simulink model "Planar_PIDC"  (R2022b)
settings: Solver=VariableStepAuto  StartTime=0.0  StopTime=40  RelTol=1e-3
values from neighbouring files (symbols this model uses):
  I = [1; 1; 1; 0.5; 0.5]*0.2    [RobDyn4link.m]
  l = [1; 1; 1; 1; 2]*0.2    [RobDyn4link.m]
  lc = l./2    [RobDyn4link.m]
  m = [1; 1; 1; 0.3; 0.3]*1    [RobDyn4link.m]
  q0 = [pi/2; -pi/4; -1*pi/6;-pi/12;0;]    [RobDyn4link.m]
  theta_max = [0.915*pi; 0.915*pi; 0.915*pi; 0.915*pi; 0.915*pi;]    [RobDyn4link.m]
  theta_min = [-0.915*pi; -0.915*pi; -0.915*pi; -0.915*pi; -0.915*pi;]    [RobDyn4link.m]
undefined symbols (not defined in the file or in its folder): DiscIntNeverNeededParam
(part 1 of 3)
settings Model: Creator=yu  LastModifiedBy=yu

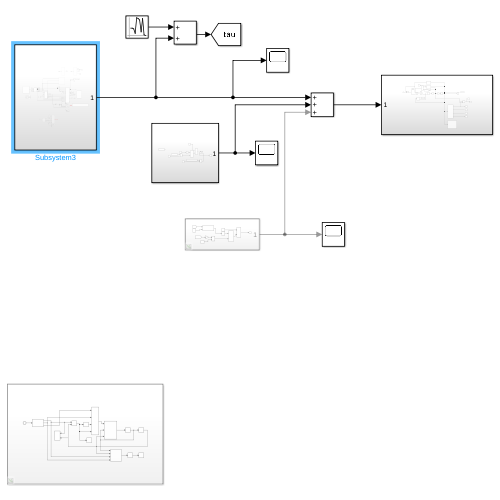
[thumbnail: Simulink's stored preview of the top-level diagram]
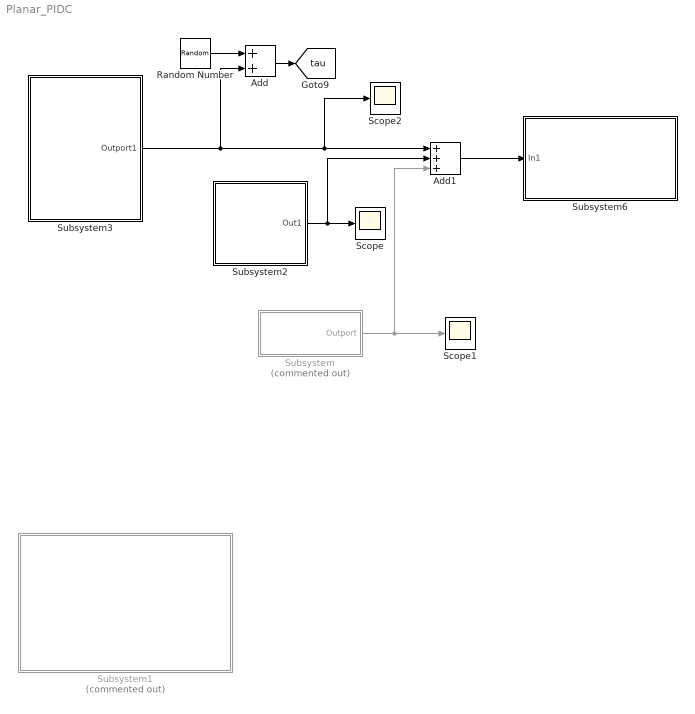
== system Planar_PIDC ==
  Add : Sum
  Add1 : Sum  Inputs=+++
  Random Number : RandomNumber  Variance=0.1
  Scope : Scope
  Scope1 : Scope
  Scope2 : Scope
  Subsystem : Subsystem  Commented=on
  Subsystem1 : Subsystem  Commented=on
  Subsystem2 : Subsystem
  Subsystem3 : Subsystem
  Subsystem6 : Subsystem
  tag scope: tau=global
  wires:
  Add1/1 -> Subsystem6/1(In1)
  Subsystem3/1(Outport1) -> Scope2/1, Add1/1, Add/2
  Subsystem2/1(Out1) -> Scope/1, Add1/2
  Subsystem/1(Outport) -> Scope1/1, Add1/3
  Random Number/1 -> Add/1
  Add/1 -> [tau]

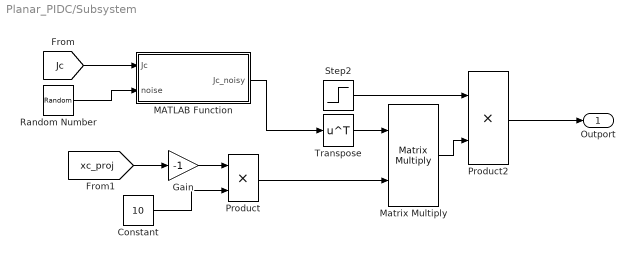
== system Planar_PIDC/Subsystem ==
  Constant : Constant  Value=10
  Gain : Gain  Gain=-1
  MATLAB Function : MATLAB Function  TreatAsAtomicUnit=on
  Matrix Multiply : Product  Multiplication=Matrix(*)
  Product : Product
  Product2 : Product
  Random Number : RandomNumber  SampleTime=0.1
  Step2 : Step  Time=5  After=5  SampleTime=0
  Transpose : Math  Operator=transpose
  Outport : Outport
  wires:
  Step2/1 -> Product2/1
  Matrix Multiply/1 -> Product2/2
  Transpose/1 -> Matrix Multiply/1
  [xc_proj] -> Gain/1
  Product/1 -> Matrix Multiply/2
  Product2/1 -> Outport/1
  [Jc] -> MATLAB Function/1(Jc)
  Constant/1 -> Product/2
  Random Number/1 -> MATLAB Function/2(noise)
  MATLAB Function/1(Jc_noisy) -> Transpose/1
  Gain/1 -> Product/1

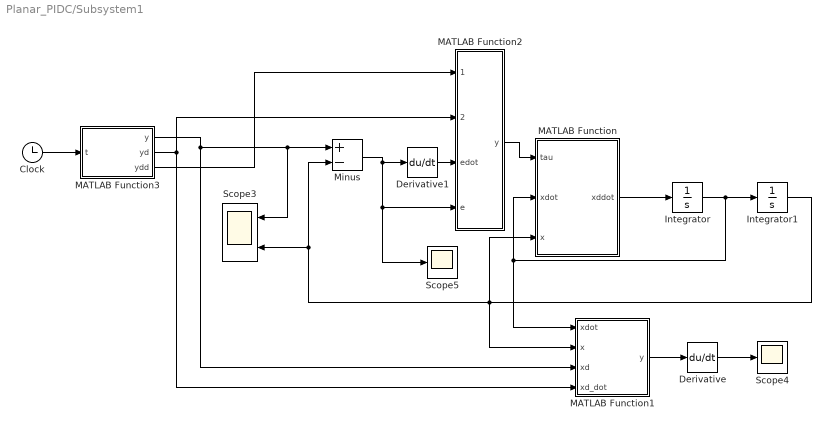
== system Planar_PIDC/Subsystem1 ==
  Clock : Clock
  Derivative : Derivative
  Derivative1 : Derivative
  Integrator : Integrator
  Integrator1 : Integrator
  MATLAB Function : MATLAB Function  TreatAsAtomicUnit=on
  MATLAB Function1 : MATLAB Function  TreatAsAtomicUnit=on
  MATLAB Function2 : MATLAB Function  TreatAsAtomicUnit=on
  MATLAB Function3 : MATLAB Function  TreatAsAtomicUnit=on
  Minus : Sum  Inputs=+-
  Scope3 : Scope  NumInputPorts=2
  Scope4 : Scope
  Scope5 : Scope
  wires:
  Derivative/1 -> Scope4/1
  MATLAB Function3/1(y) -> Scope3/1, Minus/1, MATLAB Function1/3(xd)
  MATLAB Function1/1(y) -> Derivative/1
  MATLAB Function/1(xddot) -> Integrator/1
  Integrator1/1 -> MATLAB Function1/2(x), Minus/2, Scope3/2, MATLAB Function/3(x)
  MATLAB Function2/1(y) -> MATLAB Function/1(tau)
  Clock/1 -> MATLAB Function3/1(t)
  Integrator/1 -> MATLAB Function/2(xdot), MATLAB Function1/1(xdot), Integrator1/1
  Minus/1 -> Scope5/1, MATLAB Function2/4(e), Derivative1/1
  MATLAB Function3/3(ydd) -> MATLAB Function2/1(xd_ddot)
  Derivative1/1 -> MATLAB Function2/3(edot)
  MATLAB Function3/2(yd) -> MATLAB Function2/2(xd_dot), MATLAB Function1/4(xd_dot)

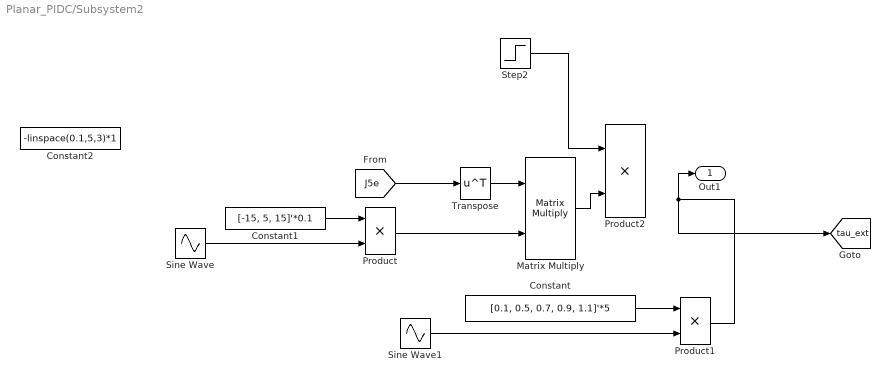
== system Planar_PIDC/Subsystem2 ==
  Constant : Constant  Value=[0.1, 0.5, 0.7, 0.9, 1.1]'*5
  Constant1 : Constant  Value=[-15, 5, 15]'*0.1
  Constant2 : Constant  Value=-linspace(0.1,5,3)*1
  Matrix Multiply : Product  Multiplication=Matrix(*)
  Product : Product
  Product1 : Product
  Product2 : Product
  Sine Wave : Sin  Frequency=0.5  SampleTime=0
  Sine Wave1 : Sin  Frequency=0.5  SampleTime=0
  Step2 : Step  Time=5  After=5  SampleTime=0
  Transpose : Math  Operator=transpose
  Out1 : Outport
  tag scope: tau_ext=global
  wires:
  [J5e] -> Transpose/1
  Transpose/1 -> Matrix Multiply/1
  Product/1 -> Matrix Multiply/2
  Matrix Multiply/1 -> Product2/2
  Product1/1 -> Out1/1, [tau_ext]
  Step2/1 -> Product2/1
  Constant1/1 -> Product/1
  Sine Wave/1 -> Product/2
  Constant/1 -> Product1/1
  Sine Wave1/1 -> Product1/2

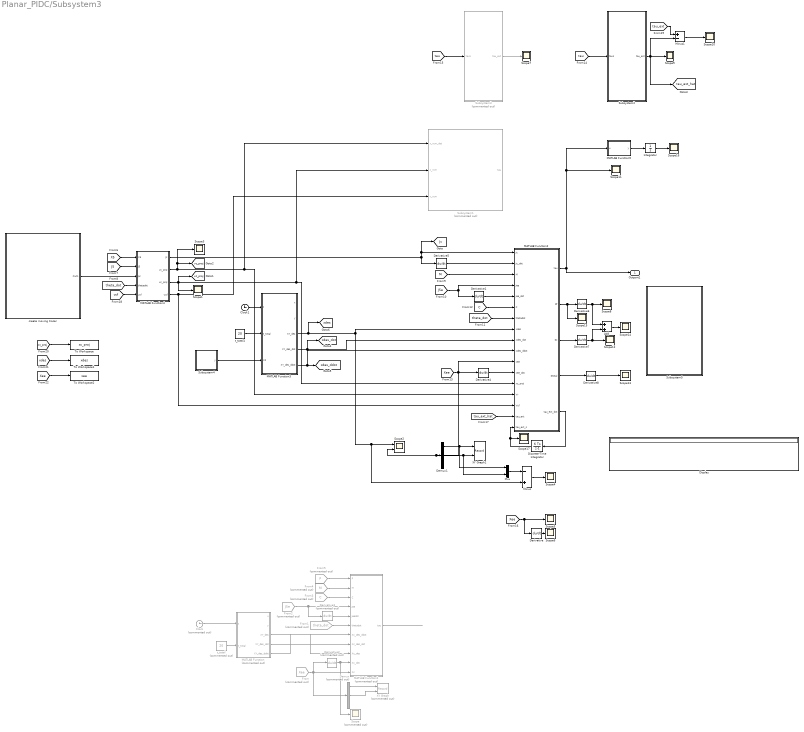
== system Planar_PIDC/Subsystem3 ==
  Add : Sum
  Clock : Clock  Commented=on
  Clock1 : Clock
  Demux : Demux  Commented=on  Outputs=3
  Demux1 : Demux  Outputs=3
  Derivative{,1,4..8} (7 alike) : Derivative
  Derivative2 : Derivative  Commented=on
  Derivative3 : Derivative  Commented=on
  Discrete-Time Integrator : DiscreteIntegrator  SampleTime=1e-3  ICPrevOutput=DiscIntNeverNeededParam  ICPrevScaledInput=DiscIntNeverNeededParam
  Display : Display
  From : From  Commented=on  GotoTag=Xee  TagVisibility=global
  From1 : From  Commented=on  GotoTag=theta_dot  TagVisibility=global
  From2 : From  Commented=on  GotoTag=J5e  TagVisibility=global
  From3 : From  Commented=on  GotoTag=C  TagVisibility=global
  From4 : From  Commented=on  GotoTag=M  TagVisibility=global
  From5 : From  Commented=on  GotoTag=P  TagVisibility=global
  Integrator : Integrator
  MATLAB Function : MATLAB Function  Commented=on  TreatAsAtomicUnit=on
  MATLAB Function1 : MATLAB Function  Commented=on  TreatAsAtomicUnit=on
  MATLAB Function2 : MATLAB Function  TreatAsAtomicUnit=on
  MATLAB Function3 : MATLAB Function  TreatAsAtomicUnit=on
  MATLAB Function4 : MATLAB Function  TreatAsAtomicUnit=on
  MATLAB Function5 : MATLAB Function  TreatAsAtomicUnit=on
  Minus : Sum  Inputs=-+
  Minus1 : Sum  Inputs=+-
  Mux : Mux  Inputs=2
  Scope : Scope  Commented=on
  Scope{1,3..17} (16 alike) : Scope
  Scope2 : Scope  NumInputPorts=2
  Subsystem1 : Subsystem  Commented=on
  Subsystem2 : Subsystem
  Subsystem3 : Subsystem  Commented=on
  Subsystem4 : Subsystem
  Subsystem5 : Subsystem
  To Workspace : ToWorkspace  VariableName=xc_proj  SaveFormat=Timeseries  SampleTime=-1
  To Workspace1 : ToWorkspace  VariableName=xdes  SaveFormat=Timeseries  SampleTime=-1
  To Workspace2 : ToWorkspace  VariableName=xee  SaveFormat=Timeseries  SampleTime=-1
  XY Graph : Record  Commented=on  FileSettingsInternal="{\"entries\":[{\"content\":{\"excelSettings\":{\"content\":{},\"type\":\"Streamout.ExcelSettings\"}},\"type\":\"Streamout.FileSettingStorage\",\"uuid\":\"\"}],\"packageUris\":[\"http:\\/\\/schema.mathworks.com\\/mf0\\/streamout_blocks\\/R2020a\"],\"version\":\"1.0\"}"  Layout=[1 1]  SignalsInternal="{\"entries\":[{\"content\":{\"signals\":[{\"content\":{\"blockPath\":[],\"channel\":[],\"dimensions\":[1,1],\"domain\":\"\",\"lineColor\":\"#a2142f\",\"plots\":[1],\"port\":1,\"sid\":[],\"signalID\":16,\"signalName\":\"Demux:1\"},\"type\":\"RecordBlkView.Signal\",\"uuid\":\"\"},{\"content\":{\"blockPath\":[],\"channel\":[],\"dimensions\":[1,1],\"domain\":\"\",\"lineColor\":\"#139fff\",\"plots\":[1],\"port\":2,\"sid\":[],\"signalID\":19,\"signalName\":\"Demux:2\"},\"type\":\"RecordBlkView.Signal\",\"uuid\":\"\"}]},\"type\":\"RecordBlkView.InputSignals\",\"uuid\":\"\"}],\"packageUris\":[\"http:\\/\\/schema.mathworks.com\\/mf0\\/streamout_blocks\\/R2020a\"],\"version\":\"1.0\"}"  VisualizationBindings="{\"xyplotplugin\":{\"info\":[{\"series\":[{\"bindingParametersList\":[{\"parameter\":\"X-Axis\",\"signalID\":16,\"signalName\":\"Demux:1\"},{\"parameter\":\"Y-Axis\",\"signalID\":19,\"signalName\":\"Demux:2\"}],\"seriesID\":63717}],\"subplotID\":1}]}}"  CompatibilityTag=XY
  XY Graph1 : Record  FileSettingsInternal="{\"entries\":[{\"content\":{\"excelSettings\":{\"content\":{},\"type\":\"Streamout.ExcelSettings\"}},\"type\":\"Streamout.FileSettingStorage\",\"uuid\":\"\"}],\"packageUris\":[\"http:\\/\\/schema.mathworks.com\\/mf0\\/streamout_blocks\\/R2020a\"],\"version\":\"1.0\"}"  Layout=[1 1]  SignalsInternal="{\"entries\":[{\"content\":{\"signals\":[{\"content\":{\"blockPath\":[],\"channel\":[],\"dimensions\":[1,1],\"domain\":\"\",\"lineColor\":\"#a2142f\",\"plots\":[1],\"port\":1,\"sid\":[\"\"],\"signalID\":6665,\"signalName\":\"Demux1:1\"},\"type\":\"RecordBlkView.Signal\",\"uuid\":\"\"},{\"content\":{\"blockPath\":[],\"channel\":[],\"dimensions\":[1,1],\"domain\":\"\",\"lineColor\":\"#139fff\",\"plots\":[1],\"port\":2,\"sid\":[\"\"],\"signalID\":6669,\"signalName\":\"Demux1:2\"},\"type\":\"RecordBlkView.Signal\",\"uuid\":\"\"}]},\"type\":\"RecordBlkView.InputSignals\",\"uuid\":\"\"}],\"packageUris\":[\"http:\\/\\/schema.mathworks.com\\/mf0\\/streamout_blocks\\/R2020a\"],\"version\":\"1.0\"}"  VisualizationBindings="{\"xyplotplugin\":{\"info\":[{\"series\":[{\"bindingParametersList\":[{\"parameter\":\"X-Axis\",\"signalID\":6665,\"signalName\":\"Demux1:1\"},{\"parameter\":\"Y-Axis\",\"signalID\":6669,\"signalName\":\"Demux1:2\"}],\"seriesID\":65386}],\"subplotID\":1}]}}"  CompatibilityTag=XY
  create moving trocar : Subsystem
  t_total : Constant  Commented=on  Value=20
  t_total1 : Constant  Value=20
  Outport1 : Outport
  tag scope: Jc=global, tau_ext_hat=global, vc_proj=global, xc_proj=global, xdes=global, xdes_ddot=global, xdes_dot=global
  wires:
  Clock/1 -> MATLAB Function/1(t)
  t_total/1 -> MATLAB Function/2(t_total)
  MATLAB Function/5(XY_des_ddot) -> MATLAB Function1/7(Xc_des_ddot)
  From/1 -> Demux/1, Derivative2/1, MATLAB Function1/11(Xc)
  Derivative2/1 -> Scope/1, MATLAB Function1/10(Xc_dot)
  From1/1 -> MATLAB Function1/6(thetadot)
  From2/1 -> Derivative3/1, MATLAB Function1/4(Jee)
  Derivative3/1 -> MATLAB Function1/5(Jeedot)
  From3/1 -> MATLAB Function1/3(C)
  From4/1 -> MATLAB Function1/2(M)
  From5/1 -> MATLAB Function1/1(P)
  MATLAB Function1/1(tau) -> ?
  MATLAB Function/3(XY_des) -> MATLAB Function1/9(Xc_des)
  MATLAB Function/4(XY_des_dot) -> MATLAB Function1/8(Xc_des_dot)
  Demux/1 -> XY Graph/1
  Demux/2 -> XY Graph/2
  [X5] -> MATLAB Function4/1(X5)
  [theta_dot] -> MATLAB Function4/4(thetadot)
  [J5] -> MATLAB Function4/2(J5)
  [M] -> MATLAB Function2/3(M)
  Derivative1/1 -> MATLAB Function2/5(Jee_dot)
  [J5e] -> MATLAB Function2/4(Jee), Derivative1/1
  [theta_dot] -> MATLAB Function2/7(thetadot)
  [C] -> MATLAB Function2/6(C)
  [Xee] -> Derivative4/1, Scope2/2, Demux1/1, MATLAB Function2/11(xee)
  Derivative4/1 -> MATLAB Function2/12(xee_dot)
  Demux1/1 -> Mux/1, XY Graph1/1
  Demux1/2 -> Mux/2, XY Graph1/2
  MATLAB Function4/3(xc_proj) -> MATLAB Function2/13(xc_proj), Subsystem1/2(x_rcm), Scope1/1, [xc_proj]
  MATLAB Function4/2(vc_proj) -> Scope3/1, [vc_proj], MATLAB Function2/14(Vr), Subsystem1/1(x_rcm_dot)
  Mux/1 -> Minus/1
  Minus/1 -> Scope4/1
  [Xee] -> Derivative/1, Scope5/1
  Derivative/1 -> Scope6/1
  [vcf] -> MATLAB Function4/5(vcf)
  create moving trocar/1(Out1) -> MATLAB Function4/3(pc)
  Derivative5/1 -> MATLAB Function2/2(Jc_dot)
  MATLAB Function4/4(Vcf) -> Subsystem1/3(v_rcm), MATLAB Function2/15(Vcf)
  MATLAB Function4/1(Jc) -> [Jc], MATLAB Function2/1(Jc), Derivative5/1
  [tau] -> Subsystem2/1(tau1)
  Subsystem2/1(tau_ext) -> [tau_ext_hat], Scope9/1, Minus1/2
  Subsystem3/1(tau_ext) -> Scope7/1
  [tau] -> Subsystem3/1(tau1)
  MATLAB Function3/3(XY_des) -> Minus/2, Scope2/1, MATLAB Function2/8(xdes), [xdes]
  MATLAB Function3/4(XY_des_dot) -> MATLAB Function2/9(xdes_dot), [xdes_dot]
  MATLAB Function3/5(XY_des_ddot) -> MATLAB Function2/10(xdes_ddot), [xdes_ddot]
  [tau_ext_hat] -> MATLAB Function2/16(tau_ext)
  [tau_ext] -> Minus1/1
  Minus1/1 -> Scope10/1
  Clock1/1 -> MATLAB Function3/1(t)
  t_total1/1 -> MATLAB Function3/2(t_total)
  Subsystem4/1(y) -> MATLAB Function3/3(X0)
  MATLAB Function2/2(Sf) -> Scope15/1, Derivative6/1
  MATLAB Function2/3(Sc) -> Derivative7/1
  Derivative6/1 -> Add/1, Scope8/1
  Derivative7/1 -> Add/2, Scope12/1
  MATLAB Function2/4(Stotal) -> Derivative8/1
  Derivative8/1 -> Scope13/1
  Add/1 -> Scope14/1
  MATLAB Function2/1(tau) -> Outport1/1, Scope11/1, MATLAB Function5/1(u)
  MATLAB Function5/1(y) -> Integrator/1
  Integrator/1 -> Scope16/1
  [xc_proj] -> To Workspace/1
  [xdes] -> To Workspace1/1
  [Xee] -> To Workspace2/1
  Discrete-Time Integrator/1 -> Scope17/1, MATLAB Function2/17(tau_ext_s)
  MATLAB Function2/5(tau_ext_dot) -> Discrete-Time Integrator/1

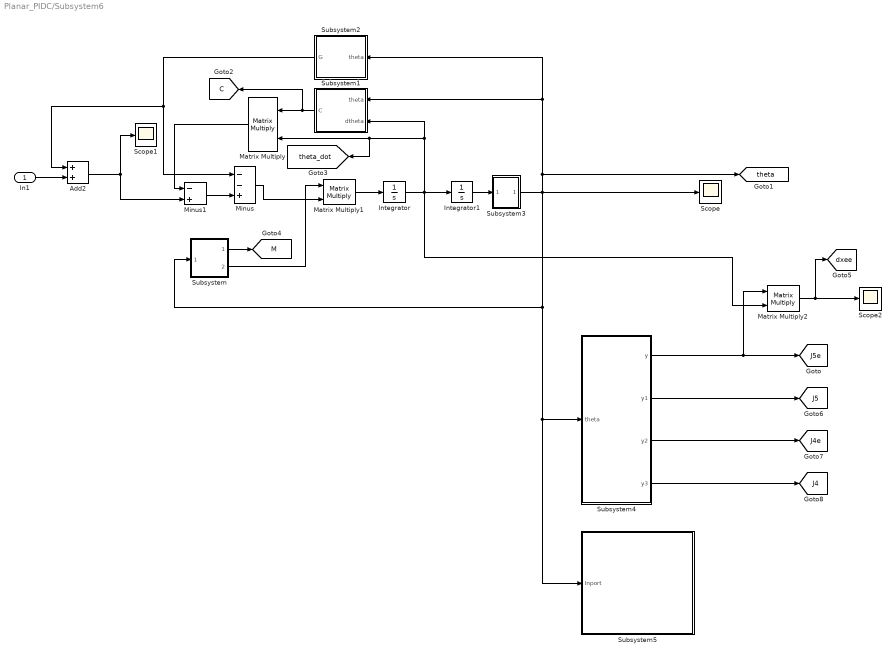
== system Planar_PIDC/Subsystem6 ==
  In1 : Inport
  Add2 : Sum
  Integrator : Integrator
  Integrator1 : Integrator  InitialCondition=q0
  Matrix Multiply : Product  Multiplication=Matrix(*)
  Matrix Multiply1 : Product  Multiplication=Matrix(*)
  Matrix Multiply2 : Product  Multiplication=Matrix(*)
  Minus : Sum  Inputs=--+
  Minus1 : Sum  Inputs=-+
  Scope : Scope
  Scope1 : Scope
  Scope2 : Scope
  Subsystem : Subsystem
  Subsystem1 : Subsystem
  Subsystem2 : Subsystem
  Subsystem3 : Subsystem
  Subsystem4 : Subsystem
  Subsystem5 : Subsystem
  tag scope: C=global, J4=global, J4e=global, J5=global, J5e=global, M=global, dxee=global, theta=global, theta_dot=global
  wires:
  Subsystem2/1(G) -> Minus/1, Add2/1
  Subsystem/2(Outport1) -> Matrix Multiply1/1
  Subsystem/1(Outport) -> [M]
  In1/1 -> Add2/2
  Integrator1/1 -> Subsystem3/1(In1)
  Integrator/1 -> Matrix Multiply2/2, Integrator1/1, Subsystem1/2(dtheta), Matrix Multiply/2, [theta_dot]
  Subsystem4/2(y1) -> [J5]
  Subsystem4/4(y3) -> [J4]
  Matrix Multiply/1 -> Minus1/1
  Add2/1 -> Minus1/2, Scope1/1
  Subsystem4/3(y2) -> [J4e]
  Subsystem3/1(theta) -> Subsystem4/1(theta), Subsystem5/1(Inport), Subsystem/1(Inport), Subsystem1/1(theta), Subsystem2/1(theta), [theta], Scope/1
  Matrix Multiply1/1 -> Integrator/1
  Subsystem4/1(y) -> [J5e], Matrix Multiply2/1
  Subsystem1/1(C) -> [C], Matrix Multiply/1
  Minus/1 -> Matrix Multiply1/2
  Matrix Multiply2/1 -> Scope2/1, [dxee]
  Minus1/1 -> Minus/3

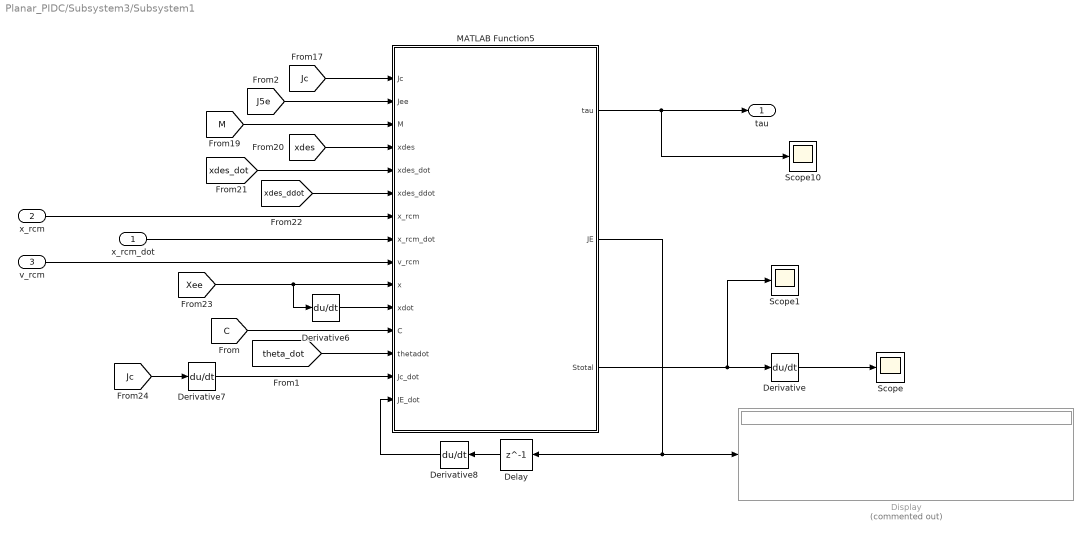
== system Planar_PIDC/Subsystem3/Subsystem1 ==
  x_rcm_dot : Inport
  x_rcm : Inport  Port=2
  v_rcm : Inport  Port=3
  Delay : Delay  DelayLength=1
  Derivative{,6..8} (4 alike) : Derivative
  Display : Display  Commented=on
  MATLAB Function5 : MATLAB Function  TreatAsAtomicUnit=on
  Scope : Scope
  Scope1 : Scope
  Scope10 : Scope
  tau : Outport
  wires:
  [xdes_dot] -> MATLAB Function5/5(xdes_dot)
  [Jc] -> MATLAB Function5/1(Jc)
  [xdes_ddot] -> MATLAB Function5/6(xdes_ddot)
  Derivative6/1 -> MATLAB Function5/11(xdot)
  v_rcm/1 -> MATLAB Function5/9(v_rcm)
  x_rcm/1 -> MATLAB Function5/7(x_rcm)
  [theta_dot] -> MATLAB Function5/13(thetadot)
  x_rcm_dot/1 -> MATLAB Function5/8(x_rcm_dot)
  Derivative7/1 -> MATLAB Function5/14(Jc_dot)
  Derivative8/1 -> MATLAB Function5/15(JE_dot)
  [C] -> MATLAB Function5/12(C)
  [Xee] -> Derivative6/1, MATLAB Function5/10(x)
  [xdes] -> MATLAB Function5/4(xdes)
  [Jc] -> Derivative7/1
  [M] -> MATLAB Function5/3(M)
  MATLAB Function5/2(JE) -> Delay/1, Display/1
  Delay/1 -> Derivative8/1
  MATLAB Function5/1(tau) -> Scope10/1, tau/1
  [J5e] -> MATLAB Function5/2(Jee)
  Derivative/1 -> Scope/1
  MATLAB Function5/3(Stotal) -> Scope1/1, Derivative/1

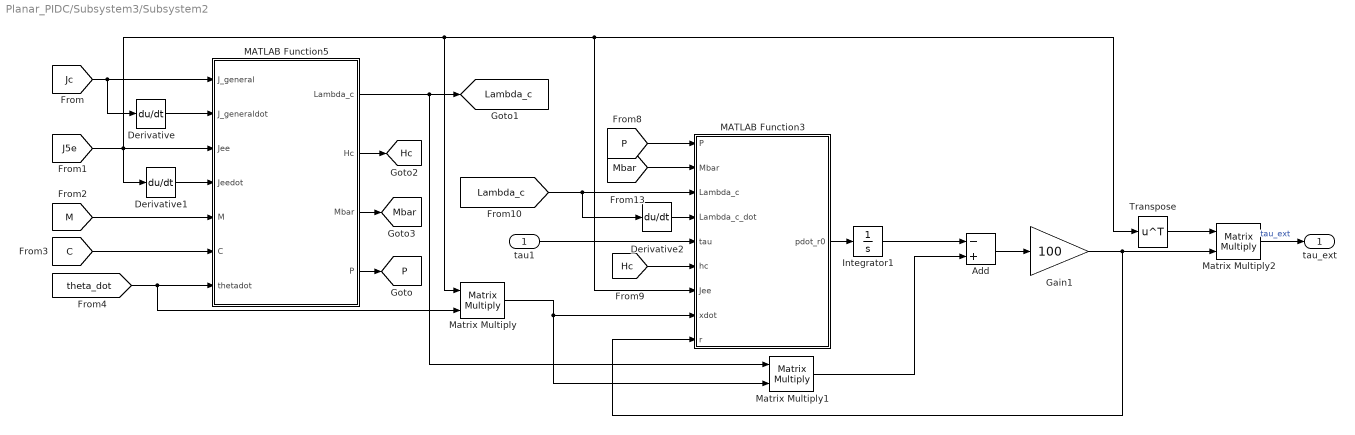
== system Planar_PIDC/Subsystem3/Subsystem2 ==
  tau1 : Inport
  Add : Sum  Inputs=-+
  Derivative : Derivative
  Derivative1 : Derivative
  Derivative2 : Derivative
  Gain1 : Gain  Gain=100
  Integrator1 : Integrator
  MATLAB Function3 : MATLAB Function  TreatAsAtomicUnit=on
  MATLAB Function5 : MATLAB Function  TreatAsAtomicUnit=on
  Matrix Multiply : Product  Multiplication=Matrix(*)
  Matrix Multiply1 : Product  Multiplication=Matrix(*)
  Matrix Multiply2 : Product  Multiplication=Matrix(*)
  Transpose : Math  Operator=transpose
  tau_ext : Outport
  tag scope: Hc=global, Lambda_c=global, Mbar=global, P=global
  wires:
  Matrix Multiply1/1 -> Add/2
  Derivative1/1 -> MATLAB Function5/4(Jeedot)
  MATLAB Function5/1(Lambda_c) -> [Lambda_c], Matrix Multiply1/1
  Gain1/1 -> Matrix Multiply2/2, MATLAB Function3/9(r)
  [J5e] -> MATLAB Function3/7(Jee), Transpose/1, Matrix Multiply/1, MATLAB Function5/3(Jee), Derivative1/1
  tau1/1 -> MATLAB Function3/5(tau)
  MATLAB Function5/2(Hc) -> [Hc]
  Matrix Multiply2/1 -> tau_ext/1  "tau_ext"
  [Lambda_c] -> Derivative2/1, MATLAB Function3/3(Lambda_c)
  Derivative/1 -> MATLAB Function5/2(J_generaldot)
  Integrator1/1 -> Add/1
  MATLAB Function3/1(pdot_r0) -> Integrator1/1
  [C] -> MATLAB Function5/6(C)
  [Hc] -> MATLAB Function3/6(hc)
  MATLAB Function5/3(Mbar) -> [Mbar]
  Matrix Multiply/1 -> MATLAB Function3/8(xdot), Matrix Multiply1/2
  Derivative2/1 -> MATLAB Function3/4(Lambda_c_dot)
  MATLAB Function5/4(P) -> [P]
  [Mbar] -> MATLAB Function3/2(Mbar)
  [P] -> MATLAB Function3/1(P)
  Transpose/1 -> Matrix Multiply2/1
  [theta_dot] -> Matrix Multiply/2, MATLAB Function5/7(thetadot)
  [Jc] -> Derivative/1, MATLAB Function5/1(J_general)
  [M] -> MATLAB Function5/5(M)
  Add/1 -> Gain1/1

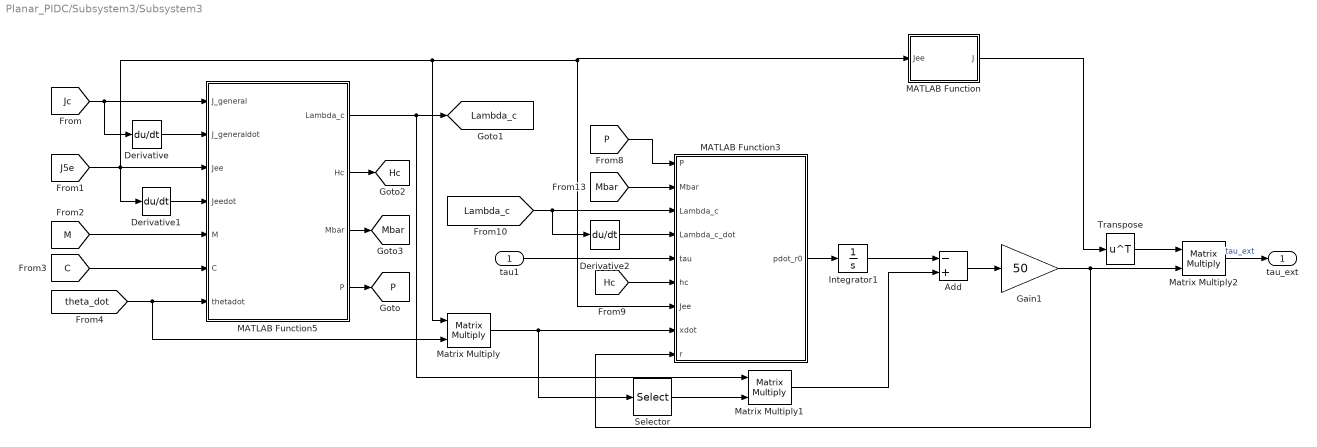
== system Planar_PIDC/Subsystem3/Subsystem3 ==
  tau1 : Inport
  Add : Sum  Inputs=-+
  Derivative : Derivative
  Derivative1 : Derivative
  Derivative2 : Derivative
  Gain1 : Gain  Gain=50
  Integrator1 : Integrator
  MATLAB Function : MATLAB Function  TreatAsAtomicUnit=on
  MATLAB Function3 : MATLAB Function  TreatAsAtomicUnit=on
  MATLAB Function5 : MATLAB Function  TreatAsAtomicUnit=on
  Matrix Multiply : Product  Multiplication=Matrix(*)
  Matrix Multiply1 : Product  Multiplication=Matrix(*)
  Matrix Multiply2 : Product  Multiplication=Matrix(*)
  Selector : Selector  InputPortWidth=3  IndexOptions=Index vector (dialog)  Indices=[1 2]  OutputSizes=1
  Transpose : Math  Operator=transpose
  tau_ext : Outport
  tag scope: Hc=global, Lambda_c=global, Mbar=global, P=global
  wires:
  Add/1 -> Gain1/1
  [M] -> MATLAB Function5/5(M)
  [Jc] -> MATLAB Function5/1(J_general), Derivative/1
  [theta_dot] -> MATLAB Function5/7(thetadot), Matrix Multiply/2
  Transpose/1 -> Matrix Multiply2/1
  [P] -> MATLAB Function3/1(P)
  [Mbar] -> MATLAB Function3/2(Mbar)
  MATLAB Function5/4(P) -> [P]
  Derivative2/1 -> MATLAB Function3/4(Lambda_c_dot)
  Matrix Multiply/1 -> Selector/1, MATLAB Function3/8(xdot)
  MATLAB Function5/3(Mbar) -> [Mbar]
  [Hc] -> MATLAB Function3/6(hc)
  [C] -> MATLAB Function5/6(C)
  MATLAB Function3/1(pdot_r0) -> Integrator1/1
  Integrator1/1 -> Add/1
  Derivative/1 -> MATLAB Function5/2(J_generaldot)
  [Lambda_c] -> MATLAB Function3/3(Lambda_c), Derivative2/1
  Matrix Multiply2/1 -> tau_ext/1  "tau_ext"
  MATLAB Function5/2(Hc) -> [Hc]
  tau1/1 -> MATLAB Function3/5(tau)
  [J5e] -> Derivative1/1, MATLAB Function5/3(Jee), Matrix Multiply/1, MATLAB Function3/7(Jee), MATLAB Function/1(Jee)
  Gain1/1 -> MATLAB Function3/9(r), Matrix Multiply2/2
  MATLAB Function5/1(Lambda_c) -> Matrix Multiply1/1, [Lambda_c]
  Derivative1/1 -> MATLAB Function5/4(Jeedot)
  Matrix Multiply1/1 -> Add/2
  MATLAB Function/1(J) -> Transpose/1
  Selector/1 -> Matrix Multiply1/2

== system Planar_PIDC/Subsystem3/Subsystem4 ==
  Clock2 : Clock
  Constant : Constant  Value=[4.673;1.966]
  Constant1 : Constant  Value=[0.9346,0.3932]
  Display : Display
  MATLAB Function5 : MATLAB Function  TreatAsAtomicUnit=on
  Memory : Memory
  y : Outport
  wires:
  Clock2/1 -> MATLAB Function5/2(t)
  [Xee] -> MATLAB Function5/1(Xee)
  Memory/1 -> MATLAB Function5/3(y_prev)
  Constant1/1 -> Memory/1, Display/1, y/1

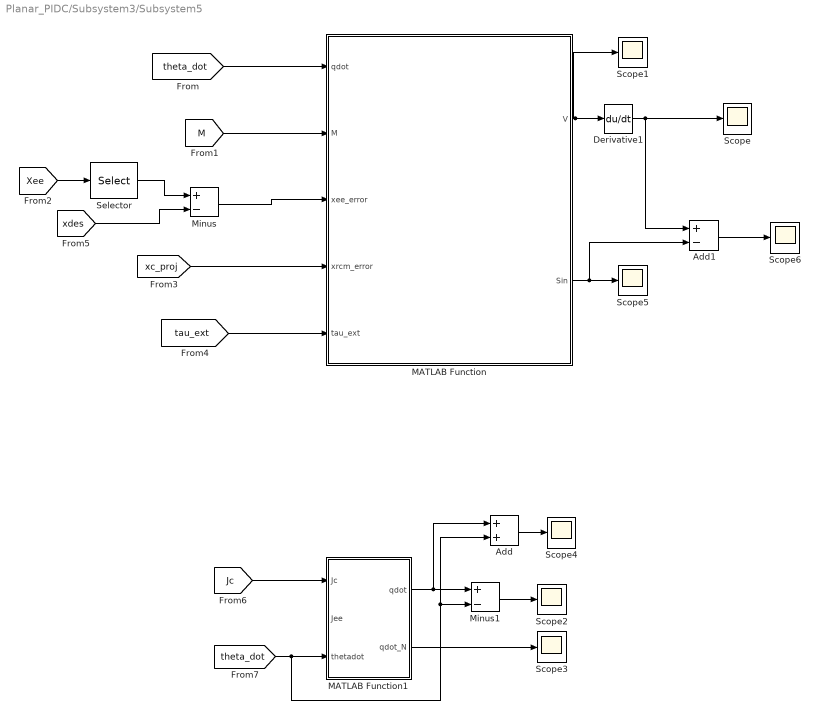
== system Planar_PIDC/Subsystem3/Subsystem5 ==
  Add : Sum
  Add1 : Sum  Inputs=+-
  Derivative1 : Derivative
  MATLAB Function : MATLAB Function  TreatAsAtomicUnit=on
  MATLAB Function1 : MATLAB Function  TreatAsAtomicUnit=on
  Minus : Sum  Inputs=+-
  Minus1 : Sum  Inputs=+-
  Scope{,1..6} (7 alike) : Scope
  Selector : Selector  InputPortWidth=3  IndexOptions=Index vector (dialog)  Indices=[1 2]  OutputSizes=1
  wires:
  [theta_dot] -> MATLAB Function/1(qdot)
  [M] -> MATLAB Function/2(M)
  [xc_proj] -> MATLAB Function/4(xrcm_error)
  [tau_ext] -> MATLAB Function/5(tau_ext)
  Minus/1 -> MATLAB Function/3(xee_error)
  MATLAB Function/1(V) -> Scope1/1, Derivative1/1
  Derivative1/1 -> Add1/1, Scope/1
  Selector/1 -> Minus/1
  [xdes] -> Minus/2
  [Xee] -> Selector/1
  [theta_dot] -> Add/2, Minus1/2, MATLAB Function1/3(thetadot)
  [Jc] -> MATLAB Function1/1(Jc)
  MATLAB Function1/1(qdot) -> Add/1, Minus1/1
  Minus1/1 -> Scope2/1
  MATLAB Function1/2(qdot_N) -> Scope3/1
  Add/1 -> Scope4/1
  MATLAB Function/2(Sin) -> Add1/2, Scope5/1
  Add1/1 -> Scope6/1

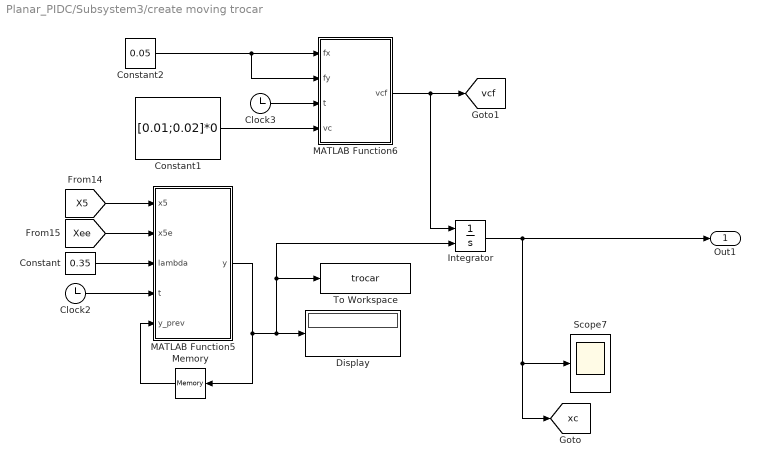
== system Planar_PIDC/Subsystem3/create moving trocar ==
  Clock2 : Clock
  Clock3 : Clock
  Constant : Constant  Value=0.35
  Constant1 : Constant  Value=[0.01;0.02]*0
  Constant2 : Constant  Value=0.05
  Display : Display
  Integrator : Integrator  InitialConditionSource=external
  MATLAB Function5 : MATLAB Function  TreatAsAtomicUnit=on
  MATLAB Function6 : MATLAB Function  TreatAsAtomicUnit=on
  Memory : Memory
  Scope7 : Scope
  To Workspace : ToWorkspace  VariableName=trocar  SaveFormat=Timeseries  SampleTime=-1
  Out1 : Outport
  tag scope: vcf=global, xc=global
  wires:
  Clock3/1 -> MATLAB Function6/3(t)
  [Xee] -> MATLAB Function5/2(x5e)
  Constant2/1 -> MATLAB Function6/2(fy), MATLAB Function6/1(fx)
  Clock2/1 -> MATLAB Function5/4(t)
  [X5] -> MATLAB Function5/1(x5)
  Constant1/1 -> MATLAB Function6/4(vc)
  MATLAB Function6/1(vcf) -> [vcf], Integrator/1
  Constant/1 -> MATLAB Function5/3(lambda)
  Integrator/1 -> Out1/1, [xc], Scope7/1
  Memory/1 -> MATLAB Function5/5(y_prev)
  MATLAB Function5/1(y) -> Memory/1, To Workspace/1, Integrator/2, Display/1

== system Planar_PIDC/Subsystem6/Subsystem ==
  Inport : Inport  PortDimensions=[5,1]
  Constant : Constant  Value=l
  Constant1 : Constant  Value=lc
  Constant2 : Constant  Value=I
  Constant3 : Constant  Value=m
  MATLAB Function : MATLAB Function  TreatAsAtomicUnit=on
  Outport : Outport  PortDimensions=[5,5]
  Outport1 : Outport  Port=2  PortDimensions=[5,5]
  wires:
  Constant3/1 -> MATLAB Function/5(m)
  MATLAB Function/1(M) -> Outport/1  "M"
  Inport/1 -> MATLAB Function/1(theta)  "theta"
  Constant2/1 -> MATLAB Function/4(I)
  Constant/1 -> MATLAB Function/2(l)
  Constant1/1 -> MATLAB Function/3(lc)
  MATLAB Function/2(Minv) -> Outport1/1  "Minv"

== system Planar_PIDC/Subsystem6/Subsystem1 ==
  theta : Inport  PortDimensions=[5,1]
  dtheta : Inport  Port=2  PortDimensions=[5,1]
  Constant : Constant  Value=m
  Constant1 : Constant  Value=l
  Constant2 : Constant  Value=lc
  MATLAB Function : MATLAB Function  TreatAsAtomicUnit=on
  C : Outport  PortDimensions=[5,5]
  wires:
  theta/1 -> MATLAB Function/1(theta)
  MATLAB Function/1(C) -> C/1
  dtheta/1 -> MATLAB Function/2(dtheta)
  Constant/1 -> MATLAB Function/3(m)
  Constant2/1 -> MATLAB Function/5(lc)
  Constant1/1 -> MATLAB Function/4(l)

== system Planar_PIDC/Subsystem6/Subsystem2 ==
  theta : Inport  PortDimensions=[5,1]
  Constant : Constant  Value=m
  Constant1 : Constant  Value=l
  Constant2 : Constant  Value=lc
  MATLAB Function : MATLAB Function  TreatAsAtomicUnit=on
  G : Outport  PortDimensions=[5,1]
  wires:
  Constant1/1 -> MATLAB Function/3(l)
  Constant2/1 -> MATLAB Function/4(lc)
  Constant/1 -> MATLAB Function/2(m)
  MATLAB Function/1(G) -> G/1
  theta/1 -> MATLAB Function/1(theta)

== system Planar_PIDC/Subsystem6/Subsystem3 ==
  In1 : Inport
  Atan2 : Trigonometry  Operator=atan2
  Constant : Constant  Value=theta_max
  Constant1 : Constant  Value=theta_min
  MATLAB Function : MATLAB Function  TreatAsAtomicUnit=on
  Sin : Trigonometry
  Sin1 : Trigonometry  Operator=cos
  theta : Outport  PortDimensions=[5,1]
  wires:
  Atan2/1 -> MATLAB Function/1(theta)
  In1/1 -> Sin1/1, Sin/1
  Sin/1 -> Atan2/1
  Sin1/1 -> Atan2/2
  MATLAB Function/1(y) -> theta/1
  Constant/1 -> MATLAB Function/2(theta_max)
  Constant1/1 -> MATLAB Function/3(theta_min)

== system Planar_PIDC/Subsystem6/Subsystem4 ==
  theta : Inport
  Constant : Constant  Value=l
  MATLAB Function : MATLAB Function  TreatAsAtomicUnit=on
  y : Outport
  y1 : Outport  Port=2
  y2 : Outport  Port=3
  y3 : Outport  Port=4
  wires:
  theta/1 -> MATLAB Function/1(theta)  "theta"
  MATLAB Function/1(J5e) -> y/1  "J5e"
  Constant/1 -> MATLAB Function/2(l)
  MATLAB Function/2(J5) -> y1/1  "J5"
  MATLAB Function/3(J4e) -> y2/1  "J4e"
  MATLAB Function/4(J4) -> y3/1  "J4"

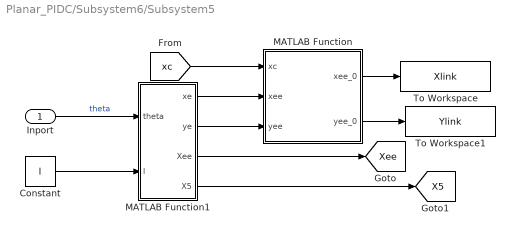
== system Planar_PIDC/Subsystem6/Subsystem5 ==
  Inport : Inport
  Constant : Constant  Value=l
  MATLAB Function : MATLAB Function  TreatAsAtomicUnit=on
  MATLAB Function1 : MATLAB Function  TreatAsAtomicUnit=on
  To Workspace : ToWorkspace  VariableName=Xlink  SaveFormat=Timeseries  SampleTime=-1
  To Workspace1 : ToWorkspace  VariableName=Ylink  SaveFormat=Timeseries  SampleTime=-1
  tag scope: X5=global, Xee=global
  wires:
  MATLAB Function1/1(xe) -> MATLAB Function/2(xee)
  MATLAB Function1/2(ye) -> MATLAB Function/3(yee)
  Inport/1 -> MATLAB Function1/1(theta)  "theta"
  Constant/1 -> MATLAB Function1/2(l)
  MATLAB Function1/3(Xee) -> [Xee]
  MATLAB Function/1(xee_0) -> To Workspace/1
  MATLAB Function/2(yee_0) -> To Workspace1/1
  MATLAB Function1/4(X5) -> [X5]
  [xc] -> MATLAB Function/1(xc)

== matlab function Planar_PIDC/Subsystem6/Subsystem3/MATLAB Function ==
  data: theta input; y output; theta_max input; theta_min input
function y = fcn(theta, theta_max, theta_min)
y= max(theta_min,min(theta, theta_max));

== matlab function Planar_PIDC/Subsystem3/MATLAB Function3 ==
  data: x output; t input; y output; t_total input; XY_des output; XY_des_dot output; XY_des_ddot output; X0 input
function [x,y,XY_des,XY_des_dot,XY_des_ddot]= fcn(t, t_total, X0)
% x0 = 0.934607;
% y0 = 0.393185;

x0 = X0(1);
y0 = X0(2);



radius = 0.05;     % Total duration to complete the circle (seconds)
% dt = 0.01;        % Time step for simulation

% Calculate center of the circle
xc = x0 - radius;
yc = y0;

omega = 2 * pi / t_total;

% Circle trajectory
x = xc + radius * cos(omega * t);
y = yc + radius * sin(omega * t);

% Velocity
xdot = -radius * omega * sin(omega * t);
ydot = radius * omega * cos(omega * t);

% Acceleration
xddot = -radius * omega^2 * cos(omega * t);
yddot = -radius * omega^2 * sin(omega * t);

XY_des = [x;y];
XY_des_dot = [xdot;ydot];
XY_des_ddot = [xddot;yddot];

== matlab function Planar_PIDC/Subsystem3/create moving trocar/MATLAB Function5 ==
  data: x5 input; y output; x5e input; lambda input; t input; y_prev input
function y = fcn(x5,x5e,lambda,t,y_prev)
if t == 0
    xc = lambda*(x5e - x5) + x5;
    y = xc(1:2);
else 
    y = y_prev;
end

== matlab function Planar_PIDC/Subsystem3/create moving trocar/MATLAB Function6 ==
  data: fx input; vcf output; fy input; t input; vc input
function vcf = fcn(fx,fy,t,vc)

vcf = [vc(1)*sin(2*pi*fx*t);
    vc(2)*cos(2*pi*fy*t)];

== matlab function Planar_PIDC/Subsystem3/Subsystem5/MATLAB Function1 ==
  data: Jc input; qdot output; Jee input; thetadot input; qdot_N output
function [qdot,qdot_N]= fcn(Jc,Jee,thetadot)
Jc_pinv = Jc'/(Jc*Jc');
P = eye(5) - Jc_pinv*Jc;
qdot = P*thetadot;
qdot_N = (eye(5) - P)*thetadot;

== matlab function Planar_PIDC/Subsystem3/Subsystem1/MATLAB Function5 ==
  data: Jc input; Jee input; tau output; M input; xdes input; xdes_dot input; xdes_ddot input; x_rcm input; x_rcm_dot input; v_rcm input; x input; xdot input; C input; thetadot input; Jc_dot input; JE_dot input; JE output; Stotal output
function [tau,JE,Stotal]= fcn(Jc,Jee,M,xdes,xdes_dot,xdes_ddot,x_rcm,x_rcm_dot, v_rcm,x,xdot,C,thetadot,Jc_dot,JE_dot)
Jm = Jc(:,1:1);
Jr = Jc(:,2:5);
Z = [-Jr'*inv(Jm)', eye(4)]';
% Z = Z;
Z_sharp = inv(Z'*M*Z)*Z'*M;

Lambda_rcm = inv(Jc/M*Jc');
Lambda_f = Z'*M*Z;
Lambda_E = zeros(5,5);
Lambda_E(1,1) = Lambda_rcm;
Lambda_E(2:5,2:5) = Lambda_f;

JE = [Jc;Z_sharp];

H_E = Lambda_E*(JE/M*C*thetadot - JE_dot*thetadot);

Kp_rcm = 100;
Kd_rcm = sqrt(2)*Kp_rcm;
Frcm = Lambda_rcm * 0 - Kd_rcm*x_rcm_dot - Kp_rcm*x_rcm - v_rcm;

xdes_aug = [xdes];
xdes_dot_aug = [xdes_dot];
xdes_ddot_aug = [xdes_ddot];

Kp = 100;
Kd = sqrt(2)*Kp;
% Kp_matrix = zeros(4,4);
% Kp_matrix(1:2,1:2) = eye(2)*Kp;
Kp_matrix = eye(2)*Kp;
% Kd_matrix = zeros(4,4);
% Kd_matrix(1:2,1:2) = eye(2)*Kd;
Kd_matrix = eye(2)*Kd;

x_aug = [x(1:2)];
xdot_aug = [xdot(1:2)];

Jee = Jee(1:2,:);
Ff =  Lambda_f(1:2,1:2)*xdes_ddot_aug +  Kd_matrix*(xdes_dot_aug - xdot_aug) + Kp_matrix*(xdes_aug - x_aug);
Ff = Z'*Jee'*Ff;

% JE = [Jc; Z_sharp];
tau = JE'*([Frcm;Ff] + H_E);

S = 0.5*((xdes_dot_aug - xdot_aug)'*Lambda_f(1:2,1:2)*(xdes_dot_aug - xdot_aug) + x_rcm_dot'*Lambda_rcm*x_rcm_dot);
V = 0.5*((xdes_aug - x_aug)'*Kp_matrix*(xdes_aug - x_aug) + x_rcm'*Kp_rcm*x_rcm);
Stotal = S + V;

== matlab function Planar_PIDC/Subsystem3/Subsystem4/MATLAB Function5 ==
  data: Xee input; y output; t input; y_prev input
function y = fcn(Xee,t,y_prev)
x0 = zeros(2,1);
if t == 0
    x0 = Xee(1:2);
    y = x0(1:2);
else 
    y = y_prev;
end

== matlab function Planar_PIDC/Subsystem3/MATLAB Function4 ==
  data: X5 input; J5 input; Jc output; vc_proj output; pc input; xc_proj output; thetadot input; vcf input; Vcf output
function [Jc,vc_proj,xc_proj,Vcf] = fcn(X5, J5, pc,thetadot,vcf)
pr = X5(1:2);
theta5 = X5(3);

R = [cos(theta5), -sin(theta5); sin(theta5), cos(theta5)];
y = R(:,2);
dir = pr - pc;
% A = [-y(1), y(2), dir(2)*y(2) - dir(1)*y(1)];
A = [-sin(theta5),cos(theta5),-cos(theta5)*dir(1) - sin(theta5)*dir(2)];
Jc = A*J5;

vc_proj = Jc*thetadot;
xc_proj = R(:,2)'*dir;

Vcf = A(:,1:2)*vcf;

== matlab function Planar_PIDC/Subsystem3/MATLAB Function ==
  data: x output; t input; y output; t_total input; XY_des output; XY_des_dot output; XY_des_ddot output
function [x,y,XY_des,XY_des_dot,XY_des_ddot]= fcn(t, t_total)
x0 = 0.934607;
y0 = 0.393185;

radius = 0.05;     % Total duration to complete the circle (seconds)
% dt = 0.01;        % Time step for simulation

% Calculate center of the circle
xc = x0 - radius;
yc = y0;

omega = 2 * pi / t_total;

% Circle trajectory
x = xc + radius * cos(omega * t);
y = yc + radius * sin(omega * t);

% Velocity
xdot = -radius * omega * sin(omega * t);
ydot = radius * omega * cos(omega * t);

% Acceleration
xddot = -radius * omega^2 * cos(omega * t);
yddot = -radius * omega^2 * sin(omega * t);

XY_des = [x;y];
XY_des_dot = [xdot;ydot];
XY_des_ddot = [xddot;yddot];

== matlab function Planar_PIDC/Subsystem3/MATLAB Function1 ==
  data: P input; tau output; M input; C input; Jee input; Jeedot input; thetadot input; Xc_des_ddot input; Xc_des_dot input; Xc_des input; Xc_dot input; Xc input
function tau = fcn(P, M, C, Jee, Jeedot, thetadot, Xc_des_ddot, Xc_des_dot, Xc_des, Xc_dot, Xc)

% Compute pseudo-inverse of Jee
Jee_pinv = Jee' / (Jee * Jee');

% Compute Lambda_x_inv
Lambda_x_inv = Jee * M^-1 * Jee';

% Gains
D_x = eye(3) * 50; 
D_x(3, 3) = 0; 
K_x = eye(3) * 100; 
K_x(3, 3) = 0;
Xc_des_ddot = [Xc_des_ddot;0];
Xc_des_dot = [Xc_des_dot;0];
Xc_des = [Xc_des;0];
% Compute desired task-space accelerations
Xdes_ddot = Xc_des_ddot + Lambda_x_inv * (D_x * (Xc_des_dot - Xc_dot) + K_x * (Xc_des - Xc));

% Compute desired joint accelerations
qdes_ddot = Jee_pinv * (Xdes_ddot - Jeedot * thetadot);

% Compute W^(-1/2)
% W = eye(5);
% [U, D] = eig(W);
% if any(diag(D) <= 0)
%     error('Matrix W must be positive definite or positive semi-definite.');
% end
% D_inv_sqrt = diag(1 ./ sqrt(max(diag(D), eps)));
% W_inv_sqrt = U * D_inv_sqrt * U';
% 
% % Compute PW_pinv and P_Winv
% PW_pinv = W_inv_sqrt / (P * W_inv_sqrt * (P * W_inv_sqrt)');
% P_Winv = W_inv_sqrt * PW_pinv;
% 
% % Compute control torque
% tau = P_Winv * P * (M * qdes_ddot + C * thetadot);
% 
% % Ensure tau is real
% assert(isreal(tau), 'Output tau must be real.');
P_pinv = P/(P*P' + 1e-3*eye(5));
tau = P*(M * qdes_ddot + C * thetadot);
end

== matlab function Planar_PIDC/Subsystem3/Subsystem5/MATLAB Function ==
  data: qdot input; V output; M input; xee_error input; xrcm_error input; tau_ext input; Sin output
function [V,Sin]= fcn(qdot,M,xee_error,xrcm_error,tau_ext)
xee_error = xee_error(1:2);
Kpee = eye(2)*10;
Kpc = 10;
V = 0.5*(qdot'*M*qdot + xee_error'*Kpee*xee_error + xrcm_error'*Kpc*xrcm_error);

Sin = qdot'*tau_ext;

== matlab function Planar_PIDC/Subsystem3/Subsystem2/MATLAB Function3 ==
  data: P input; Mbar input; Lambda_c input; Lambda_c_dot input; pdot_r0 output; tau input; hc input; Jee input; xdot input; r input
function pdot_r0 = fcn(P,Mbar,Lambda_c,Lambda_c_dot,tau,hc,Jee,xdot,r)
% Jee_pinv = Jee'/(Jee*Jee' + 0*eye(3));
% F = Jee_pinv'*tau;

F = Lambda_c*Jee/Mbar*P*tau;
pdot_r0 = Lambda_c_dot*xdot + F - hc + r;

== matlab function Planar_PIDC/Subsystem/MATLAB Function ==
  data: Jc input; Jc_noisy output; noise input
function Jc_noisy = fcn(Jc, noise)
Kn = 0.01;
Jc_noisy = Jc + ones(1,5)*noise*Kn;

== matlab function Planar_PIDC/Subsystem3/Subsystem3/MATLAB Function3 ==
  data: P input; Mbar input; Lambda_c input; Lambda_c_dot input; pdot_r0 output; tau input; hc input; Jee input; xdot input; r input
function pdot_r0 = fcn(P,Mbar,Lambda_c,Lambda_c_dot,tau,hc,Jee,xdot,r)
% Jee_pinv = Jee'/(Jee*Jee' + 0*eye(3));
% F = Jee_pinv'*tau;
Jee = Jee(1:2,:);
xdot = xdot(1:2);
F = Lambda_c*Jee/Mbar*P*tau;
pdot_r0 = Lambda_c_dot*xdot + F - hc + r;

== matlab function Planar_PIDC/Subsystem3/Subsystem3/MATLAB Function5 ==
  data: Lambda_c output size=[2,2]; Hc output; J_general input; J_generaldot input; Jee input; Jeedot input; M input; C input; thetadot input; Mbar output; P output
function [Lambda_c,Hc,Mbar,P] = fcn(J_general,J_generaldot,Jee,Jeedot,M,C,thetadot)
Jc = J_general;
Jc_pinv = Jc'/(Jc*Jc' + 0*eye(1));
P = eye(5) - Jc_pinv*Jc;

%% previous part
% Pnull = eye(5) - P;
% Mc = P*M + (eye(5) - P);
% Lambda_c = (Jee * (Mc \ P) * Jee'+ 1e-3*eye(3) ) \ eye(3);
% 
% PMP = P*M*P;
% McInvP = PMP'*(PMP*PMP');
% % Lambda_c = eye(3)/(Jee*McInvP*Jee'+1e-1*eye(3));
% 
% coder.extrinsic('computeLambdaC');
% Lambda_c = eye(3);
% Lambda_c = computeLambdaC(Jee,Mc,P,1e-6);

%% Farhad Aghili 2016 ICRA
nv = 0.5;
Mbar = P*M*P + nv*(eye(5) - P);
S = eye(5) - M/Mbar*P;
Jcdot = J_generaldot;
Gamma = -Jc_pinv*Jcdot;
Omega = Gamma - Gamma';

coder.extrinsic('svdInverse');
Lambda_c = eye(2);

Jee = Jee(1:2,:);
Jeedot = Jeedot(1:2,:);

Lambda_c = svdInverse(Jee*(Mbar \ P)*Jee',1e-4);
% Lambda_c = (Jee*(Mbar \ P)*Jee' + 1e-2*eye(3)) \ eye(3);

Hc = Lambda_c*(Jee/Mbar*(Mbar*S'*Omega*thetadot + P*C*thetadot) - Jeedot*thetadot);

== matlab function Planar_PIDC/Subsystem3/Subsystem3/MATLAB Function ==
  data: Jee input; J output
function J = fcn(Jee)

J = Jee(1:2,:);

== matlab function Planar_PIDC/Subsystem1/MATLAB Function ==
  data: tau input; xddot output; xdot input; x input
function xddot = fcn(tau,xdot, x)

m = 5;
D = 1;
xddot = 1/m*(tau - D*xdot);
